simulink model "dc_motor_model"  (Simulink 7.4)
settings: Solver=ode15s  StartTime=0.0  StopTime=3  MaxStep=1e-2  RelTol=1e-3
libraries: fl_lib x10, nesl_utility x4, dspsnks4 x3, elec_lib x1
Description:
  | Linear Electric Actuator (Motor Model)
  | 
  | This model shows how to model a linear actuator.  It consists
  | of a DC motor driving a 6.25:1 worm gear which in turn drives a 3mm
  | lead screw to produce linear motion. Manufacturer data for the
  | actuator defines no-load linear speed (26mm/s), rated load (1000N),
  | rated-load linear speed (19mm/s), and maximum current (5A). The
  | maximum static force is 4000N and the rated voltage is 24V DC.
  | 
  | If friction and rotor damping are neglected, the DC Motor mask
  | parameters can be  calculated as follows. A no-load speed of 26mm/s
  | is equivalent to (26/3)*6.25*60=3250rpm. The rated motor speed is
  | (19/3)*6.25*60=2375rpm, and the rated power is
  | 1000N*19e-3m/s=19W. To run the model based on these parameters,
  | set the DC Motor Model parameterization parameter to By rated
  | power, rated speed & no-load speed and remove the Friction block.
  | The results validate the speeds for zero and 1000N load, but
  | under-predict the maximum current and maximum static force.
  | 
  | For a more accurate approximation of the motor, friction effects
  | must be included. The no-load and rated-load speed information
  | depends on the unknown friction levels, so instead we parameterize
  | the motor in terms of the maximum current which occurs when the
  | rotor is locked (i.e. no  back emf). Then the winding resistance is
  | given by rated voltage divided by maximum current i.e. 24V/5A = 4.8
  | ohms. The torque constant is given by maximum static torque divided
  | by the current i.e. (4000N*3e-3m/s/(2*pi*6.25))/4.8A = 0.3056Nm/A.
  | To run the model based on these parameters, set the DC Motor
  | Model Parameterization parameter to By equivalent circuit parameters
  | and reinstate the Friction block. You should find that a torsional friction
  | of 0.03Nm results in a 26mm/s no-load speed. The model also
  | confirms rated-load speed is 19mm/s, maximum current is 5A and
  | maximum linear force is 4000N.
  | 
  | Note that a limitation of this model is that the load can back drive
  | the motor through the worm gear. A more detailed friction
  | model would be required to prevent this.
  | 
  | 
  | 
  | 
  | Copyright 2008-2009 The MathWorks(TM), Inc.
settings Model: Creator=rhyde  LastModifiedBy=Owner  ExtModeAutoUpdateStatusClock=off
settings SolverCC: ZeroCrossControl=EnableAll
settings DataIOCC: ExternalInput=[Col_trq, brkwy_trq]  SaveTime=off
settings OptimizationCC: InitFltsAndDblsToZero=on
settings DebuggingCC: SaveWithParameterizedLinksMsg=none  SignalResolutionControl=TryResolveAllWithWarning
settings GRTTargetCC: TargetFcnLib=ansi_tfl_tmw.mat
settings SimEventsCC: propDiagAttribOutput=1  propDiagFcnCallOutput=1  propDiagStatOutput=0

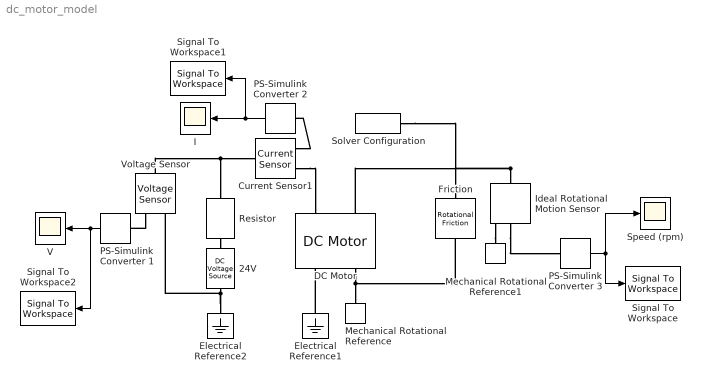
== system dc_motor_model ==
  24V : fl_lib/Electrical/Electrical Sources/DC Voltage Source  DialogController=NetworkEngine.DynNeDlgSource  SystemSampleTime=-1  v0=24 V  i_Log=off  v_Log=off  LocalVarNames=|current|voltage|power  LocalVarDescs=|Current (A)|Voltage (V)|Power (W)  LocalVarLogging=[0 0 0]
  Current Sensor1 : fl_lib/Electrical/Electrical Sensors/Current Sensor  DialogController=NetworkEngine.DynNeDlgSource  SystemSampleTime=-1  i1_Log=off  v1_Log=off  LocalVarNames=|i1|v1  LocalVarDescs=|i1|v1  LocalVarLogging=[0 0]
  DC Motor : elec_lib/Actuators & Drivers/DC Motor  DialogController=NetworkEngine.DynNeDlgSource  SystemSampleTime=-1  parameterization=1  Ra=4.8 Ohm  La=1600e-6 H  emf_or_torque=2  Kv=0.0637 V/rpm  Ki=0.0637 N*m/A  T_stall=3e-3*4000/(2*pi*6.25) N*m  w_max=3250 rpm  w_rated=2375 rpm  P_rated=19 W  V_rated=24 V  J=2.5e-5 kg*m^2  lam=1e-08 N*m/(rad/s)  speed0=0 rpm  current_Log=off  voltage_Log=off  power_Log=off  i2r_Log=off  torque_Log=off  speed_Log=off  LocalVarNames=|current|voltage|power|i2r|torque|speed  LocalVarDescs=|Current (A)|Voltage (V)|Power (W)|Electrical losses (W)|Torque (Nm)|Angular speed (rad/s)  LocalVarLogging=[0 0 0 0 0 0]
  Electrical Reference1 : fl_lib/Electrical/Electrical Elements/Electrical Reference  DialogController=NetworkEngine.DynNeDlgSource  SystemSampleTime=-1  i_Log=off  LocalVarNames=|i  LocalVarDescs=|i  LocalVarLogging=[]
  Electrical Reference2 : fl_lib/Electrical/Electrical Elements/Electrical Reference  DialogController=NetworkEngine.DynNeDlgSource  SystemSampleTime=-1  i_Log=off  LocalVarNames=|i  LocalVarDescs=|i  LocalVarLogging=[]
  Friction : fl_lib/Mechanical/Rotational Elements/Rotational Friction  DialogController=NetworkEngine.DynNeDlgSource  SystemSampleTime=-1  brkwy_trq=3.0e-2 N*m  Col_trq=3.0e-2 N*m  visc_coef=0 N*m/(rad/s)  trans_coef=10 s/rad  vel_thr=0.1 rad/s  t_Log=off  w_Log=off  LocalVarNames=|friction_torque|rel_velocity|power  LocalVarDescs=|Friction torque (N*m)|Relative velocity (rad/s)|Power (W)  LocalVarLogging=[0 0 0]
  I : Scope
      settings: YMin=-100  YMax=100
  Ideal Rotational Motion Sensor : fl_lib/Mechanical/Mechanical Sensors/Ideal Rotational Motion Sensor  DialogController=NetworkEngine.DynNeDlgSource  SystemSampleTime=-1  offset=0 rad  w_Log=off  t_Log=off  phi_Log=off  LocalVarNames=|w|t|phi  LocalVarDescs=|w|t|phi  LocalVarLogging=[]
  Mechanical Rotational Reference : fl_lib/Mechanical/Rotational Elements/Mechanical Rotational Reference  DialogController=NetworkEngine.DynNeDlgSource  SystemSampleTime=-1  t_Log=off  LocalVarNames=|t  LocalVarDescs=|t  LocalVarLogging=[]
  Mechanical Rotational Reference1 : fl_lib/Mechanical/Rotational Elements/Mechanical Rotational Reference  DialogController=NetworkEngine.DynNeDlgSource  SystemSampleTime=-1  t_Log=off  LocalVarNames=|t  LocalVarDescs=|t  LocalVarLogging=[]
  PS-Simulink Converter 1 : nesl_utility/PS-Simulink Converter  DialogController=NetworkEngine.DynNeUtilDlgSource  SystemSampleTime=-1  PhysicalDomain=network_engine_domain  LeftPortType=input  RightPortType=output  SubClassName=ps_output  Unit=V  AffineConversion=off
  PS-Simulink Converter 2 : nesl_utility/PS-Simulink Converter  DialogController=NetworkEngine.DynNeUtilDlgSource  SystemSampleTime=-1  PhysicalDomain=network_engine_domain  LeftPortType=input  RightPortType=output  SubClassName=ps_output  Unit=A  AffineConversion=off
  PS-Simulink Converter 3 : nesl_utility/PS-Simulink Converter  DialogController=NetworkEngine.DynNeUtilDlgSource  SystemSampleTime=-1  PhysicalDomain=network_engine_domain  LeftPortType=input  RightPortType=output  SubClassName=ps_output  Unit=rpm  AffineConversion=off
  Resistor : fl_lib/Electrical/Electrical Elements/Resistor  DialogController=NetworkEngine.DynNeDlgSource  SystemSampleTime=-1  R=3 Ohm  i_Log=off  v_Log=off  LocalVarNames=|i|v  LocalVarDescs=|i|v  LocalVarLogging=[0 0]
  Signal To Workspace : dspsnks4/Signal To Workspace  SystemSampleTime=-1  VariableName=rpm_motor  FrameMode=Concatenate frames (2-D array)
      settings: MaxDataPoints=1  FixptAsFi=off
  Signal To Workspace1 : dspsnks4/Signal To Workspace  SystemSampleTime=-1  VariableName=i_motor  FrameMode=Concatenate frames (2-D array)
      settings: MaxDataPoints=1  FixptAsFi=off
  Signal To Workspace2 : dspsnks4/Signal To Workspace  SystemSampleTime=-1  VariableName=v_motor  FrameMode=Concatenate frames (2-D array)
      settings: MaxDataPoints=1  FixptAsFi=off
  Solver Configuration : nesl_utility/Solver Configuration  DialogController=NetworkEngine.DynNeUtilDlgSource  SystemSampleTime=-1  PhysicalDomain=network_engine_domain  LeftPortType=input  RightPortType=generic  SubClassName=solver  Accelerate=off  Profile=off  Reg=off  Der=off  ResidualTolerance=1e-9  MaxNonlinIter=12  MaxModeIter=2  DoFixedCost=off  DoDC=off  LinearAlgebra=Sparse  LocalSolverSampleTime=.001  LocalSolverChoice=NE_BACKWARD_EULER_ADVANCER  UseLocalSolver=off
  Speed (rpm) : Scope
      settings: YMin=-500  YMax=4500  SaveName=ScopeData3
  V : Scope
      settings: YMin=-100  YMax=100
  Voltage Sensor : fl_lib/Electrical/Electrical Sensors/Voltage Sensor  DialogController=NetworkEngine.DynNeDlgSource  SystemSampleTime=-1  i1_Log=off  v1_Log=off  LocalVarNames=|i1|v1  LocalVarDescs=|i1|v1  LocalVarLogging=[0 0]
  wires:
  PS-Simulink Converter 2/1 -> I/1, Signal To Workspace1/1
  PS-Simulink Converter 1/1 -> V/1, Signal To Workspace2/1
  PS-Simulink Converter 3/1 -> Speed (rpm)/1, Signal To Workspace/1
  connections:
  DC Motor/RConn2 -- Mechanical Rotational Reference/LConn1 -- Friction/RConn1
  Ideal Rotational Motion Sensor/LConn1 -- DC Motor/LConn2 -- Friction/LConn1 -- Solver Configuration/RConn1
  Current Sensor1/RConn2 -- DC Motor/LConn1
  Current Sensor1/RConn1 -- PS-Simulink Converter 2/LConn1
  Voltage Sensor/LConn1 -- Current Sensor1/LConn1 -- Resistor/LConn1
  24V/RConn1 -- Voltage Sensor/RConn2 -- Electrical Reference2/LConn1
  Electrical Reference1/LConn1 -- DC Motor/RConn1
  Voltage Sensor/RConn1 -- PS-Simulink Converter 1/LConn1
  Resistor/RConn1 -- 24V/LConn1
  Ideal Rotational Motion Sensor/RConn2 -- PS-Simulink Converter 3/LConn1
  Ideal Rotational Motion Sensor/RConn1 -- Mechanical Rotational Reference1/LConn1
